simulink model "PHIL_testing"  (R2023b)
settings: Solver=ode4  StartTime=0.0  StopTime=inf  FixedStep=Ts  RelTol=1e-3
PostLoadFcn:
  | init;
InitFcn:
  | init;
values from neighbouring files (symbols this model uses):
  CURRENT_INPUT_OFFSET_PHA = 0    [init.m]
  CURRENT_INPUT_OFFSET_PHB = 0    [init.m]
  CURRENT_INPUT_OFFSET_PHC = 0    [init.m]
  CURRENT_INPUT_SCALE_PHA = 30    [init.m]
  CURRENT_INPUT_SCALE_PHB = 30    [init.m]
  CURRENT_INPUT_SCALE_PHC = 30    [init.m]
  ENABLE_PHA = 1    [init.m]
  ENABLE_PHB = 1    [init.m]
  ENABLE_PHC = 1    [init.m]
  FNOM = 60.0    (= 60)    [init.m]
  FREQUENCY = 60.0    (= 60)    [init.m]
  FREQUENCY_MAX_LIMIT = 66.0    (= 66)    [init.m]
  FREQUENCY_MIN_LIMIT = 56.0    (= 56)    [init.m]
  FRT_CONDITION = [1 1 1 0 ]    [init.m]
  FRT_END_TIMING = [0.2 0.3 0.4 0.5]    [init.m]
  FRT_START_TIMING = [0.1 0.2 0.3 0.4]    [init.m]
  FRT_VALUES = [59.0 56.0 55.0 33.0]    [init.m]
  MODE = 1    [init.m]
  PCRT_CONDITION = [ 0    1     0     2     0     3      0      4      0      4      0   ]    [init.m]
  PCRT_END_TIMING = [30.0 30.32 60.32 60.64 90.64 90.96 120.96 175.96 205.96 260.96 290.96]    [init.m]
  PCRT_START_TIMING = [ 0.0 30.0  30.32 60.32 60.64 90.64  90.96 120.96 175.96 205.96 260.96]    [init.m]
  PCRT_VALUES = [ 0.0 60.0   0.0  60.0   0.0  60.0    0.0   20.0    0.0  340.0    0.0 ]    [init.m]
  PHASE = [0.0 -120.0 120.0]    [init.m]
  PHNOM = [0 -120 120]    [init.m]
  Pnom = 5e3    (= 5000)    [init.m]
  RMS_ENABLE = 0    [init.m]
  ROCOF_ENABLE = 0    [init.m]
  ROCOF_INIT = 60    [init.m]
  ROCOF_VALUE = 3    [init.m]
  ROCOM_ENABLE = 1    [init.m]
  ROCOM_END_TIME = 100    [init.m]
  ROCOM_INIT = 1    [init.m]
  ROCOM_START_TIME = 0    [init.m]
  ROCOM_VALUE = 13.8    [init.m]
  Srated = 5e3    (= 5000)    [init.m]
  Ts = 40e-6    (= 4e-05)    [init.m]
  VNOM = 1.0    (= 1)    [init.m]
  VOLT_INPUT_OFFSET_PHA = 0    [init.m]
  VOLT_INPUT_OFFSET_PHB = 0    [init.m]
  VOLT_INPUT_OFFSET_PHC = 0    [init.m]
  VOLT_INPUT_SCALE_PHA = 100    [init.m]
  VOLT_INPUT_SCALE_PHB = 100    [init.m]
  VOLT_INPUT_SCALE_PHC = 100    [init.m]
  VOLT_OUTPUT_SCALE_PHA = 5.6    [init.m]
  VOLT_OUTPUT_SCALE_PHB = 5.6    [init.m]
  VOLT_OUTPUT_SCALE_PHC = 5.6    [init.m]
  VOLTAGE = [1.0 1.0 1.0]    [init.m]
  VOLTAGE_MAX_LIMIT = 1.1    [init.m]
  VOLTAGE_MIN_LIMIT = 0.0    (= 0)    [init.m]
  VRT_CONDITION = [0 1 0 1 0 1 0 1 -1 -1 -1 -1 -1 -1 -1 -1 -1 -1 -1 -1]+1    [init.m]
  VRT_END_TIMING = [0.2 0.3 0.4 0.5 0.6 0.7 0.8 0.9 1 1.1 1.2 1.3 1.4 1.5 1.6 1.7 1.8 1.9 2 2.1]    [init.m]
  VRT_PHA_ENABLE = 0    [init.m]
  VRT_PHB_ENABLE = 0    [init.m]
  VRT_PHC_ENABLE = 0    [init.m]
  VRT_START_TIMING = [0.1 0.2 0.3 0.4 0.5 0.6 0.7 0.8 0.9 1 0.1 0.2 0.3 0.4 0.5 0.6 0.7 0.8 0.9 1]    [init.m]
  VRT_VALUES = [1.2 0.94 0 0.5 0.7 0.88 0.94 0.88 0.94 1.1 1.2 0.94 0 0.5 0.7 0.88 0.94 0.88 0.94 1.1]    [init.m]
  WAV_ENABLE = 1    [init.m]
undefined symbols (not defined in the file or in its folder): another_event_name, DiscIntNeverNeededParam, EX, magnitude, my_event_name, TE0741_4, TwoSSS_AIO_CPWM
libraries: simulink x14, rtlab x6, simulink_extras x6, spsRMSLib x6, rtio_opalrt_common x4, eePowerMeasurement x3, rtio_opalrt_ml605ex1 x2, spsPLL3phLib x1, spspowerguiLib x1
(part 1 of 2)
settings Model: ARTEMISmethode_block_infos=$$__separator__$$  NumberOfSteps=10  Creator=DETLDAQ  LastModifiedBy=eudesjar
settings SolverCC: AlgebraicLoopSolver=TrustRegion
settings DataIOCC: LimitDataPoints=on  SaveFormat=Array  ReturnWorkspaceOutputs=off
settings OptimizationCC: BlockReduction=off  BooleanDataType=off  OptimizeBlockIOStorage=off  BufferReuse=off  GlobalBufferReuse=off  ExpressionFolding=off  LocalBlockOutputs=off  LifeSpan=inf  OptimizeDataStoreBuffers=off  BusAssignmentInplaceUpdate=off
settings DebuggingCC: SaveWithParameterizedLinksMsg=none  UnderspecifiedInitializationDetection=Classic  MergeDetectMultiDrivingBlocksExec=none  SignalResolutionControl=TryResolveAllWithWarning  MultiTaskDSMMsg=warning  MultiTaskCondExecSysMsg=none  UnconnectedInputMsg=warning  UnconnectedOutputMsg=warning  UnconnectedLineMsg=warning  StateNameClashWarn=warning  SFUnexpectedBacktrackingDiag=warning  SFNoUnconditionalDefaultTransitionDiag=warning  SFExecutionAtInitializationDiag=none  ArithmeticOperatorsInVariantConditions=warning
settings HardwareCC: ProdBitPerPointer=32  ProdBitPerSizeT=32  ProdBitPerPtrDiffT=32  ProdLargestAtomicFloat=None  ProdIntDivRoundTo=Undefined  ProdEndianess=Unspecified  ProdWordSize=32  ProdHWDeviceType=32-bit Generic  TargetBitPerPointer=64  TargetBitPerSizeT=64  TargetBitPerPtrDiffT=64  TargetLongLongMode=on  TargetIntDivRoundTo=Zero  TargetEndianess=LittleEndian  TargetWordSize=64  TargetHWDeviceType=MATLAB Host  ProdEqTarget=off
settings ModelReferenceCC: EnableRefExpFcnMdlSchedulingChecks=on  PropagateSignalLabelsOutOfModel=off
settings SFSimCC: SimUseLocalCustomCode=off  CustomCodeUndefinedFunction=UseInterfaceOnly
settings RTWCC: RTWUseLocalCustomCode=off  DLArmComputeVersion=19.05
settings CodeAppCC: StateflowObjectComments=on
settings GRTTargetCC: TargetLangStandard=C89/C90 (ANSI)
settings ConfigComp: CovMetricSettings=dw  CovSaveCumulativeToWorkspaceVar=on  CovSaveSingleToWorkspaceVar=on  CovExternalEMLEnable=off
settings SimscapeCC: SimscapeNormalizeSystem=off

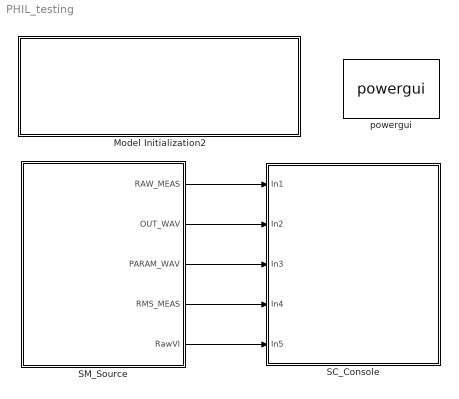
== system PHIL_testing ==
  Model Initialization2 : Subsystem  AncestorBlock=artemis/Tools /Misc/Model Initialization  mask(Model Functions){InitFcnX=init;, prel=off, posl=on, inif=on, strf=off}
      mask prompts: InitFcnX "Initialisation"; prel "Preload Function"; posl "PostLoad Function"; inif "InitFcn"; strf "StartFcn"
      mask init:
      | currentBlock = gcb;
      | root = bdroot(currentBlock);
      | 
      | if ~strcmp(get_param(root,'BlockDiagramType'),'library')
      |     if prel==1
      |         set_param(root, 'PreLoadFcn', InitFcnX);
      |     else
      |         set_param(root, 'PreLoadFcn', '');
      |     end
      |     if inif==1
      |         set_param(root, 'InitFcn', InitFcnX);
      |     else
      |         set_param(root, 'InitFcn', '');
      |     end
      |     if strf==1
      |         set_param(root, 'StartFcn', InitFcnX);
      |     else
      |         set_param(root, 'StartFcn', '');
      |     end
      |     if posl==1
      |         set_param(root, 'PostLoadFcn', InitFcnX);
      |     else
      |         set_param(root, 'PostLoadFcn', '');
      |     end
      | end
      | 
      | pos = get_param(currentBlock, 'Position');
      | width = pos(3) - pos(1); height = pos(4) - pos(2);
      | txt = [ upper(root) '\n' '- InitFcn. . . . . '  get_param(root, 'InitFcn') ];
      settings: CopyFcn=set_param(gcb,'LinkStatus','inactive')
      mask Display: text(5, height*0.5, txt, 'horizontalAlignment', 'left', 'verticalAlignment', 'middle') ;
  SC_Console : Subsystem
  SM_Source : Subsystem
  powergui : spspowerguiLib/powergui  Priority=1  SimulationMode=Discrete  SampleTime=Ts  frequency=60  Iterations=50  frequencyindice=0  Pbase=100e6  ErrMax=1e-4  UnitsV=kV  UnitsW=MW  buscounter=0  FunctionMessages=off  echomessages=off  EnableUseOfTLC=off  CurrentSourceSwitches=off  DisableSnubberDevices=off  DisableRonSwitches=off  DisableVfSwitches=off  DisplayEquations=off  AutomaticDiscreteSolvers=off  SolverType=Backward Euler  Interpol=off  ExternalGateDelay=off  methode=off  Ts=100  x0status=blocks  SPID=off  SwTol=0  HookPort=off  NonlinearTolerance=1e-4  nMaxIteration=100  ContinueOnMaxIteration=off  RestoreLinks=warning  ResistiveCurrentMeasurement=off  Frange=[0:2:500]  Ylog=off  Xlog=on  ShowGrid=off  save=off  variable=ZData  structure=0  ZoomFFT=off  StartTime=0.0  cycles=1  DisplayStyle=1  fundamental=60  FreqAxis=off  MaxFrequency=1000  frequencyindicesteady=1  RmsSteady=1  display=off
  wires:
  SM_Source/1(RAW_MEAS) -> SC_Console/1(In1)
  SM_Source/2(OUT_WAV) -> SC_Console/2(In2)
  SM_Source/3(PARAM_WAV) -> SC_Console/3(In3)
  SM_Source/4(RMS_MEAS) -> SC_Console/4(In4)
  SM_Source/5(RawVI) -> SC_Console/5(In5)

== system PHIL_testing/Model Initialization2 ==

== system PHIL_testing/SC_Console ==
  note: measurement after signal conditionning
  note: Input voltage and current after scaling and filtering
  note: Input voltage and current before scaling and filtering
  In1 : Inport
  In2 : Inport  Port=2
  In3 : Inport  Port=3
  In4 : Inport  Port=4
  In5 : Inport  Port=5
  Bus Selector : BusSelector  OutputSignals=voltage_pha,voltage_phb,voltage_phc,current_pha,current_phb,current_phc
  Bus Selector1 : BusSelector  OutputSignals=voltage_RMS,current_RMS,frequency,active_power,reactive_power,power_factor
  Bus Selector2 : BusSelector  OutputSignals=Raw Ia,Raw Ib,Raw Ic,Raw Va,Raw Vb,Raw Vc
  Display : Display
  Display1 : Display
  Display2 : Display
  Mux : Mux  Inputs=3
  Mux1 : Mux  Inputs=3
  OpComm : rtlab/OpComm  nbport=5  groupe_acq=1  subsys_rate=0  st=0  Synchronization=on  Interpolation=on  Threshold=1.0  Missed_Data=off  Sim_Time=off  Samples=off  dynSigOut=off  from_console=0  warning_done=off  writeOpCommFile=off  Offset=off
      settings: SourceProductName=RT-LAB
  Scope1 : Scope  NumInputPorts=6
  Scope2 : Scope  NumInputPorts=6
  Scope3 : Scope  NumInputPorts=3
  wires:
  In1/1 -> OpComm/1
  In2/1 -> OpComm/2
  In3/1 -> OpComm/3
  In4/1 -> OpComm/4
  OpComm/1 -> Bus Selector/1
  Bus Selector/1 -> Mux/1  "<voltage_pha>"
  Bus Selector/3 -> Mux/3  "<voltage_phc>"
  Mux/1 -> Scope3/1
  Mux1/1 -> Scope3/2
  Bus Selector/5 -> Mux1/2  "<current_phb>"
  Bus Selector/6 -> Mux1/3  "<current_phc>"
  Bus Selector/4 -> Mux1/1  "<current_pha>"
  OpComm/2 -> Scope3/3  "Output waveform"
  OpComm/3 -> Display/1  "waveform parameters"
  OpComm/4 -> Bus Selector1/1
  Bus Selector1/1 -> Display1/1, Scope1/1  "<voltage_RMS>"
  Bus Selector1/2 -> Display2/1, Scope1/2  "<current_RMS>"
  Bus Selector1/3 -> Scope1/3  "<frequency>"
  Bus Selector1/4 -> Scope1/4  "<active_power>"
  Bus Selector1/5 -> Scope1/5  "<reactive_power>"
  Bus Selector1/6 -> Scope1/6  "<power_factor>"
  In5/1 -> OpComm/5
  OpComm/5 -> Bus Selector2/1
  Bus Selector2/1 -> Scope2/1  "<Raw Ia>"
  Bus Selector2/2 -> Scope2/2  "<Raw Ib>"
  Bus Selector2/4 -> Scope2/4  "<Raw Va>"
  Bus Selector2/5 -> Scope2/5  "<Raw Vb>"
  Bus Selector2/6 -> Scope2/6  "<Raw Vc>"
  Bus Selector2/3 -> Scope2/3  "<Raw Ic>"
  Bus Selector/2 -> Mux/2  "<voltage_phb>"

== system PHIL_testing/SM_Source ==
  note: Phase, magnitude and frequency parameters of the waveform generator
  note: Voltage waveform sent as analog output
  note: RMS measurement after signal conditionning
  note: This subsytem includes a data acquistion system, a waveform generator and their control schemes
  note: This block is used to monitor the model's overruns with SVP
  note: Raw measurement before scaling and filtering
  note: Input connection with specific testbench Input blocks (needs to be redefined for new setup)
  note: Raw measurement after scaling and filtering
  note: output connection with specific testbench output blocks (needs to be redefined for new setup)
  Control : Subsystem
  InputConnections : Subsystem
  OpMonitor : rtlab/Monitoring/OpMonitor  compute_time=on  real_step=on  idle_time=on  nb_overruns=on  user_time=off  user_name=my_event_name,another_event_name
      settings: SourceProductName=RT-LAB
  OutputConnections : Subsystem
  Terminator : Terminator
  overruns : Gain
  RAW_MEAS : Outport  VectorParamsAs1DForOutWhenUnconnected=off
  OUT_WAV : Outport  Port=2  VectorParamsAs1DForOutWhenUnconnected=off
  PARAM_WAV : Outport  Port=3  VectorParamsAs1DForOutWhenUnconnected=off
  RMS_MEAS : Outport  Port=4  VectorParamsAs1DForOutWhenUnconnected=off
  RawVI : Outport  Port=5  VectorParamsAs1DForOutWhenUnconnected=off
  wires:
  InputConnections/1(RAW_MEAS (Nominal)) -> Control/1(RAW_MEAS (Nominal)), [RAW_MEAS]
  OpMonitor/4 -> overruns/1
  Control/1(OUT_WAV (PU)) -> [OUT_WAV], OutputConnections/1(OUT_WAV (PU))  "Output waveform"
  Control/2(PARAM_WAV (PU)) -> [PARAM_WAV]
  [PARAM_WAV] -> PARAM_WAV/1
  [RAW_MEAS] -> RAW_MEAS/1
  [OUT_WAV] -> OUT_WAV/1
  Control/3(RMS_MEAS) -> RMS_MEAS/1
  InputConnections/2(Out1) -> RawVI/1  "Raw measurements"
  overruns/1 -> Terminator/1

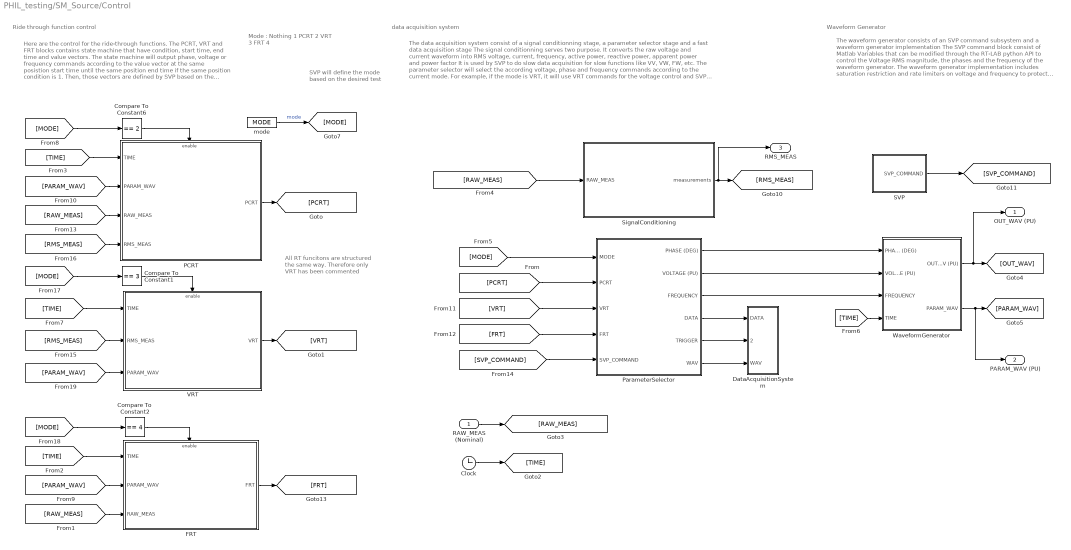
== system PHIL_testing/SM_Source/Control ==
  note: The waveform generator consists of an SVP command subsystem and a waveform generator implementation
      |
      | The SVP command block consist of Matlab Variables that can be modified through the RT-LAB python API to control the Voltage RMS magnitude, the phases and the frequency of the waveform generator.
      |
      | The waveform generator implementation includes saturation restriction and rate limiters on voltage and frequency to protect testbenches equipements. Those limits needs to be be setup properly in init.m. Then, after applying the different limitation, the voltage magnitude, phase and frequency is converted into a voltage waveform signal.
  note: The data acquisition system consist of a signal conditionning stage, a parameter selector stage and a fast data acquisition stage
      |
      | The signal conditionning serves two purpose.
      | It converts the raw voltage and current waveform into RMS voltage, current, frequency, active power, reactive power, apparent power and power factor
      | It is used by SVP to do slow data acquisition for slow functions like VV, VW, FW, etc.
      |
      | The parameter selector will select the according voltage, phase and frequency commands according to the current mode. For example, if the mode is VRT, it will use VRT commands for the voltage control and SVP commands for frequency and phase.
      |
      | The fast Data Acquisition System is used for fast recording since SVP is not fast enough to record transient behavior which is required for RT tests.
  note: All RT funcitons are structured the same way. Therefore only VRT has been commented
  note: SVP will define the mode based on the desired test
  note: Here are the control for the ride-through functions. The PCRT, VRT and FRT blocks contains state machine that have condition, start time, end time and value vectors. The state machine will output phase, voltage or frequency commands according to the value vector at the same posistion start time until the same position end time if the same position condition is 1.
      |
      | Then, those vectors are defined by SVP based on the script configuration.
  note: data acquisition system
  note: Waveform Generator
  note: Ride through function control
  note: Mode :
      |
      | Nothing
      | 1
      |
      | PCRT
      | 2
      |
      | VRT
      | 3
      |
      | FRT
      | 4
  RAW_MEAS (Nominal) : Inport
  Clock : Clock
  Compare To Constant1 : simulink/Logic and Bit Operations/Compare To Constant  relop===  const=3  OutDataTypeStr=boolean
  Compare To Constant2 : simulink/Logic and Bit Operations/Compare To Constant  relop===  const=4  OutDataTypeStr=boolean
  Compare To Constant6 : simulink/Logic and Bit Operations/Compare To Constant  relop===  const=2  OutDataTypeStr=boolean
  DataAcquisitionSystem : Subsystem
  FRT : Subsystem
  PCRT : Subsystem
  ParameterSelector : Subsystem
  SVP : Subsystem
  SignalConditioning : Subsystem
  VRT : Subsystem
  WaveformGenerator : Subsystem
  mode : Constant  Value=MODE
  OUT_WAV (PU) : Outport  VectorParamsAs1DForOutWhenUnconnected=off
  PARAM_WAV (PU) : Outport  Port=2  VectorParamsAs1DForOutWhenUnconnected=off
  RMS_MEAS : Outport  Port=3  VectorParamsAs1DForOutWhenUnconnected=off
  wires:
  mode/1 -> [MODE]  "mode"
  [RAW_MEAS] -> SignalConditioning/1(RAW_MEAS)
  [TIME] -> WaveformGenerator/4(TIME)
  ParameterSelector/5(TRIGGER) -> DataAcquisitionSystem/2(TRIGGER)
  ParameterSelector/1(PHASE (DEG)) -> WaveformGenerator/1(PHASE (DEG))
  [SVP_COMMAND] -> ParameterSelector/5(SVP_COMMAND)
  [MODE] -> ParameterSelector/1(MODE)
  Clock/1 -> [TIME]
  [MODE] -> Compare To Constant6/1
  [FRT] -> ParameterSelector/4(FRT)
  ParameterSelector/4(DATA) -> DataAcquisitionSystem/1(DATA)
  ParameterSelector/2(VOLTAGE (PU)) -> WaveformGenerator/2(VOLTAGE (PU))
  [VRT] -> ParameterSelector/3(VRT)
  WaveformGenerator/1(OUT_WAV (PU)) -> OUT_WAV (PU)/1, [OUT_WAV]
  [PCRT] -> ParameterSelector/2(PCRT)
  [RMS_MEAS] -> VRT/2(RMS_MEAS)
  ParameterSelector/3(FREQUENCY) -> WaveformGenerator/3(FREQUENCY)
  PCRT/1(PCRT) -> [PCRT]
  Compare To Constant6/1 -> PCRT/Enable
  [MODE] -> Compare To Constant1/1
  VRT/1(VRT) -> [VRT]
  [MODE] -> Compare To Constant2/1
  WaveformGenerator/2(PARAM_WAV) -> PARAM_WAV (PU)/1, [PARAM_WAV]
  Compare To Constant1/1 -> VRT/Enable
  [PARAM_WAV] -> VRT/3(PARAM_WAV)
  RAW_MEAS (Nominal)/1 -> [RAW_MEAS]
  [TIME] -> VRT/1(TIME)
  [TIME] -> FRT/1(TIME)
  Compare To Constant2/1 -> FRT/Enable
  FRT/1(FRT) -> [FRT]
  [PARAM_WAV] -> FRT/2(PARAM_WAV)
  [RAW_MEAS] -> FRT/3(RAW_MEAS)
  ParameterSelector/6(WAV) -> DataAcquisitionSystem/3(WAV)
  SignalConditioning/1(measurements) -> RMS_MEAS/1, [RMS_MEAS]
  SVP/1(SVP_COMMAND) -> [SVP_COMMAND]
  [RMS_MEAS] -> PCRT/4(RMS_MEAS)
  [PARAM_WAV] -> PCRT/2(PARAM_WAV)
  [RAW_MEAS] -> PCRT/3(RAW_MEAS)
  [TIME] -> PCRT/1(TIME)

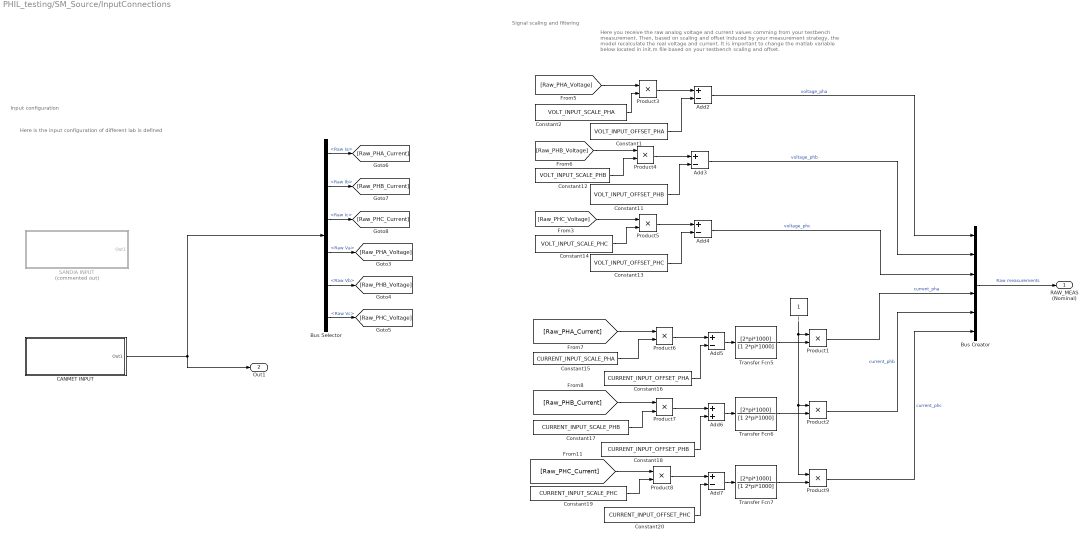
== system PHIL_testing/SM_Source/InputConnections ==
  note: Here is the input configuration of different lab is defined
  note: Input configuration
  note: Here you receive the raw analog voltage and current values comming from your testbench measurement. Then, based on scaling and offset induced by your measurement strategy, the model recalculate the real voltage and current.
      |
      | It is important to change the matlab variable below located in init.m file based on your testbench scaling and offset.
  note: Signal scaling and filtering
  Add{2..5,7} (5 alike) : Sum  Inputs=+-
  Add6 : Sum
  Bus Creator : BusCreator  Inputs=6
  Bus Selector : BusSelector  OutputSignals=Raw Ia,Raw Ib,Raw Ic,Raw Va,Raw Vb,Raw Vc
  CANMET INPUT : Subsystem
  Constant1 : Constant  Value=VOLT_INPUT_OFFSET_PHA
  Constant11 : Constant  Value=VOLT_INPUT_OFFSET_PHB
  Constant12 : Constant  Value=VOLT_INPUT_SCALE_PHB
  Constant13 : Constant  Value=VOLT_INPUT_OFFSET_PHC
  Constant14 : Constant  Value=VOLT_INPUT_SCALE_PHC
  Constant15 : Constant  Value=CURRENT_INPUT_SCALE_PHA
  Constant16 : Constant  Value=CURRENT_INPUT_OFFSET_PHA
  Constant17 : Constant  Value=CURRENT_INPUT_SCALE_PHB
  Constant18 : Constant  Value=CURRENT_INPUT_OFFSET_PHB
  Constant19 : Constant  Value=CURRENT_INPUT_SCALE_PHC
  Constant2 : Constant  Value=VOLT_INPUT_SCALE_PHA
  Constant20 : Constant  Value=CURRENT_INPUT_OFFSET_PHC
  I : Constant
  Product{1..9} (9 alike) : Product
  SANDIA INPUT : Subsystem  Commented=on
  Transfer Fcn5 : TransferFcn  Numerator=[2*pi*1000]  Denominator=[1 2*pi*1000]
  Transfer Fcn6 : TransferFcn  Numerator=[2*pi*1000]  Denominator=[1 2*pi*1000]
  Transfer Fcn7 : TransferFcn  Numerator=[2*pi*1000]  Denominator=[1 2*pi*1000]
  RAW_MEAS (Nominal) : Outport  VectorParamsAs1DForOutWhenUnconnected=off
  Out1 : Outport  Port=2  VectorParamsAs1DForOutWhenUnconnected=off
  wires:
  [Raw_PHB_Current] -> Product7/1
  Product6/1 -> Add5/1
  Constant17/1 -> Product7/2
  I/1 -> Product2/1, Product9/1, Product1/1
  Transfer Fcn6/1 -> Product2/2
  Constant14/1 -> Product5/2
  Constant13/1 -> Add4/2
  [Raw_PHB_Voltage] -> Product4/1
  Product8/1 -> Add7/1
  Product5/1 -> Add4/1
  Constant15/1 -> Product6/2
  [Raw_PHC_Voltage] -> Product5/1
  Constant20/1 -> Add7/2
  Add6/1 -> Transfer Fcn6/1
  Add5/1 -> Transfer Fcn5/1
  Product7/1 -> Add6/1
  [Raw_PHA_Voltage] -> Product3/1
  Constant18/1 -> Add6/2
  [Raw_PHA_Current] -> Product6/1
  Transfer Fcn7/1 -> Product9/2
  [Raw_PHC_Current] -> Product8/1
  Add7/1 -> Transfer Fcn7/1
  Constant16/1 -> Add5/2
  Transfer Fcn5/1 -> Product1/2
  Product4/1 -> Add3/1
  Product3/1 -> Add2/1
  Constant19/1 -> Product8/2
  Add2/1 -> Bus Creator/1  "voltage_pha"
  Add3/1 -> Bus Creator/2  "voltage_phb"
  Add4/1 -> Bus Creator/3  "voltage_phc"
  Product1/1 -> Bus Creator/4  "current_pha"
  Product2/1 -> Bus Creator/5  "current_phb"
  Product9/1 -> Bus Creator/6  "current_phc"
  Bus Creator/1 -> RAW_MEAS (Nominal)/1  "Raw measurements"
  Constant2/1 -> Product3/2
  Constant11/1 -> Add3/2
  Constant12/1 -> Product4/2
  Constant1/1 -> Add2/2
  Bus Selector/1 -> [Raw_PHA_Current]  "<Raw Ia>"
  Bus Selector/2 -> [Raw_PHB_Current]  "<Raw Ib>"
  Bus Selector/3 -> [Raw_PHC_Current]  "<Raw Ic>"
  Bus Selector/4 -> [Raw_PHA_Voltage]  "<Raw Va>"
  Bus Selector/5 -> [Raw_PHB_Voltage]  "<Raw Vb>"
  Bus Selector/6 -> [Raw_PHC_Voltage]  "<Raw Vc>"
  CANMET INPUT/1(Out1) -> Out1/1, Bus Selector/1

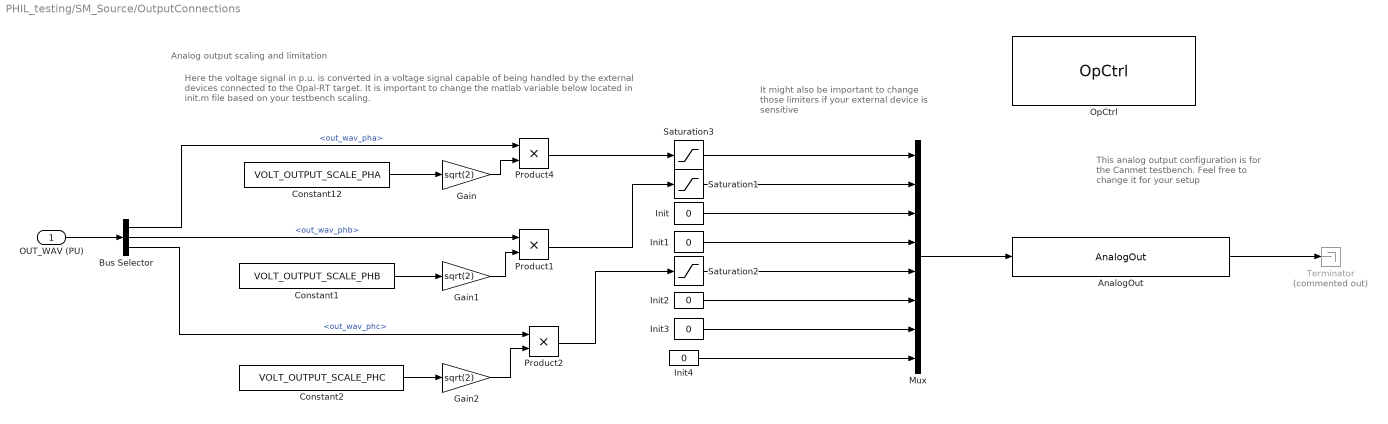
== system PHIL_testing/SM_Source/OutputConnections ==
  note: This analog output configuration is for the Canmet testbench. Feel free to change it for your setup
  note: It might also be important to change those limiters if your external device is sensitive
  note: Here the voltage signal in p.u. is converted in a voltage signal capable of being handled by the external devices connected to the Opal-RT target.
      |
      | It is important to change the matlab variable below located in init.m file based on your testbench scaling.
  note: Analog output scaling and limitation
  OUT_WAV (PU) : Inport
  AnalogOut : rtio_opalrt_common/AnalogOut  CtrlName='OpCtrl'  portNb=7  FcnNos=Slot 2 Module B Subsection 1  size=16  maxcount=8  count=8  numchan=8  israngeinput=off  voltagerange=[-16 ... 16]  slot=1  side=1  mismatch=0  slotside=Slot_2_Module_B
      settings: AttributesFormatString=%<CtrlName>  SourceProductName=RT-LAB I/O
  Bus Selector : BusSelector  OutputSignals=out_wav_pha,out_wav_phb,out_wav_phc
  Constant1 : Constant  Value=VOLT_OUTPUT_SCALE_PHB
  Constant12 : Constant  Value=VOLT_OUTPUT_SCALE_PHA
  Constant2 : Constant  Value=VOLT_OUTPUT_SCALE_PHC
  Gain : Gain  Gain=sqrt(2)
  Gain1 : Gain  Gain=sqrt(2)
  Gain2 : Gain  Gain=sqrt(2)
  Init{,1..4} (5 alike) : Constant  Value=0
  Mux : Mux  Inputs=8
  OpCtrl : rtio_opalrt_common/OpCtrl  CtrlName='OpCtrl'  boardid=0  BitstreamFilename=TE0741_4-EX-0001-3_5_0_817-TwoSSS_AIO_CPWM-04-01.bin  numconfig=-1  mode=Master  externalClock=off  decimRtsi=0  calibIO=off  SampleTime=0  loadinport=-1  BoardType=TE0741  SecondaryPresent=off  sync_type=Optical fiber  scope_enable=off  fsdFileName=TE0741_4-EX-0001-3_5_0_817-TwoSSS_AIO_CPWM-04-01.fsd  mismatch_disable=on
      settings: SourceProductName=RT-LAB I/O
  Product1 : Product
  Product2 : Product
  Product4 : Product
  Saturation1 : Saturate  UpperLimit=15  LowerLimit=-15
  Saturation2 : Saturate  UpperLimit=15  LowerLimit=-15
  Saturation3 : Saturate  UpperLimit=15  LowerLimit=-15
  Terminator : Terminator  Commented=on
  wires:
  OUT_WAV (PU)/1 -> Bus Selector/1
  Product1/1 -> Saturation1/1
  Product2/1 -> Saturation2/1
  Product4/1 -> Saturation3/1
  Constant12/1 -> Gain/1
  Bus Selector/1 -> Product4/1  "<out_wav_pha>"
  Constant1/1 -> Gain1/1
  Bus Selector/2 -> Product1/1  "<out_wav_phb>"
  Constant2/1 -> Gain2/1
  Bus Selector/3 -> Product2/1  "<out_wav_phc>"
  Saturation2/1 -> Mux/5
  Saturation3/1 -> Mux/1
  Saturation1/1 -> Mux/2
  Mux/1 -> AnalogOut/1
  Init/1 -> Mux/3
  Init1/1 -> Mux/4
  Init2/1 -> Mux/6
  Init3/1 -> Mux/7
  Init4/1 -> Mux/8
  AnalogOut/1 -> Terminator/1
  Gain/1 -> Product4/2
  Gain1/1 -> Product1/2
  Gain2/1 -> Product2/2

== system PHIL_testing/SM_Source/Control/DataAcquisitionSystem ==
  note: There is two types of recording depending on the RT function requirements either RMS or waveform data acquisition
  note: Here the RT state machine will send a trigger signal to start the recording
  DATA : Inport
  TRIGGER : Inport  Port=2
  WAV : Inport  Port=3
  Compare To Constant1 : simulink/Logic and Bit Operations/Compare To Constant  relop===  const=1  OutDataTypeStr=boolean
  Compare To Constant2 : simulink/Logic and Bit Operations/Compare To Constant  relop===  const=1  OutDataTypeStr=boolean
  Constant : Constant  Value=RMS_ENABLE
  Constant1 : Constant  Value=WAV_ENABLE
  OpTrigger : rtlab/DataLogging/OpTrigger  Trig_Type=TRIGGER SIGNAL >= TRIGGER LEVEL  Trig_Offset=-(1/Ts)  Acq_Group=28
      settings: SourceProductName=RT-LAB
  OpTrigger1 : rtlab/DataLogging/OpTrigger  Trig_Type=TRIGGER SIGNAL >= TRIGGER LEVEL  Trig_Offset=0  Acq_Group=27
      settings: SourceProductName=RT-LAB
  Subsystem : Subsystem
  Subsystem1 : Subsystem
  TRIGGER_STATUS : Gain
  TRIGGER_STATUS1 : Gain
  Terminator2 : Terminator
  Terminator3 : Terminator
  Trigger_level : Constant
  wires:
  OpTrigger/1 -> TRIGGER_STATUS/1
  Trigger_level/1 -> OpTrigger/2, OpTrigger1/2
  TRIGGER_STATUS/1 -> Terminator2/1
  TRIGGER_STATUS1/1 -> Terminator3/1
  OpTrigger1/1 -> TRIGGER_STATUS1/1
  TRIGGER/1 -> OpTrigger1/1, OpTrigger/1
  DATA/1 -> Subsystem/1(In1)
  Constant/1 -> Compare To Constant1/1
  Compare To Constant1/1 -> Subsystem/Enable
  Constant1/1 -> Compare To Constant2/1
  Compare To Constant2/1 -> Subsystem1/Enable
  WAV/1 -> Subsystem1/1(In1)

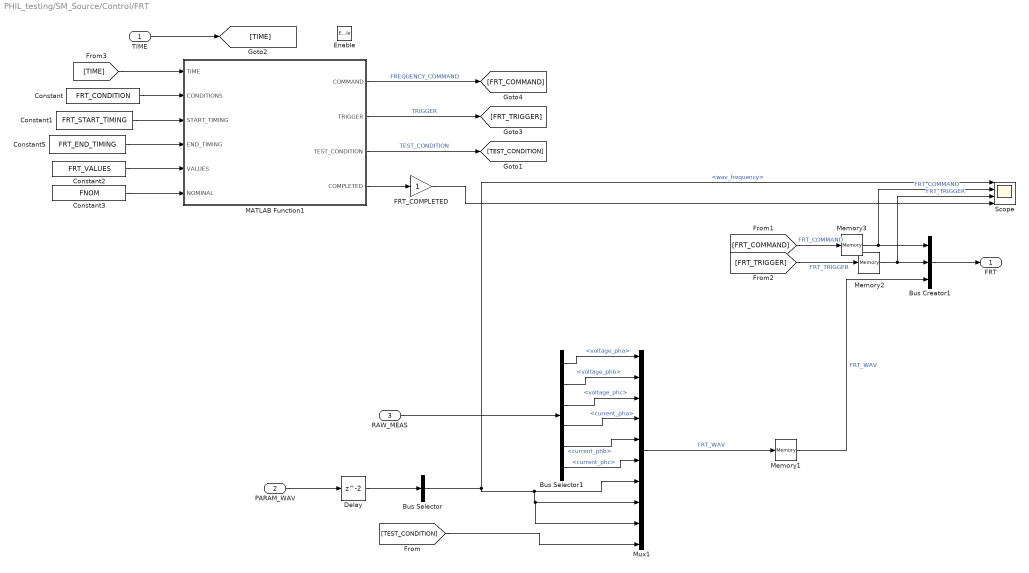
== system PHIL_testing/SM_Source/Control/FRT ==
  TIME : Inport
  PARAM_WAV : Inport  Port=2
  RAW_MEAS : Inport  Port=3
  Enable : EnablePort
  Bus Creator1 : BusCreator  Inputs=3
  Bus Selector : BusSelector  OutputSignals=wav_frequency
  Bus Selector1 : BusSelector  OutputSignals=voltage_pha,voltage_phb,voltage_phc,current_pha,current_phb,current_phc
  Constant : Constant  Value=FRT_CONDITION
  Constant1 : Constant  Value=FRT_START_TIMING
  Constant2 : Constant  Value=FRT_VALUES
  Constant3 : Constant  Value=FNOM
  Constant5 : Constant  Value=FRT_END_TIMING
  Delay : Delay
  FRT_COMPLETED : Gain
  MATLAB Function1 : MATLAB Function  TreatAsAtomicUnit=on
  Memory1 : Memory  InheritSampleTime=on  LinearizeMemory=on
  Memory2 : Memory  InheritSampleTime=on  LinearizeMemory=on
  Memory3 : Memory  InitialCondition=FNOM  InheritSampleTime=on  LinearizeMemory=on
  Mux1 : Mux  Inputs=10
  Scope : Scope  NumInputPorts=4
  FRT : Outport
  wires:
  Mux1/1 -> Memory1/1  "FRT_WAV"
  MATLAB Function1/1(COMMAND) -> [FRT_COMMAND]  "FREQUENCY_COMMAND"
  MATLAB Function1/3(TEST_CONDITION) -> [TEST_CONDITION]  "TEST_CONDITION"
  [TIME] -> MATLAB Function1/1(TIME)
  [FRT_TRIGGER] -> Memory2/1  "FRT_TRIGGER"
  Constant/1 -> MATLAB Function1/2(CONDITIONS)
  TIME/1 -> [TIME]
  Constant2/1 -> MATLAB Function1/5(VALUES)
  Constant5/1 -> MATLAB Function1/4(END_TIMING)
  MATLAB Function1/2(TRIGGER) -> [FRT_TRIGGER]  "TRIGGER"
  PARAM_WAV/1 -> Delay/1
  Bus Creator1/1 -> FRT/1
  MATLAB Function1/4(COMPLETED) -> FRT_COMPLETED/1
  Constant1/1 -> MATLAB Function1/3(START_TIMING)
  [FRT_COMMAND] -> Memory3/1  "FRT_COMMAND"
  [TEST_CONDITION] -> Mux1/10
  Delay/1 -> Bus Selector/1
  Bus Selector/1 -> Scope/1, Mux1/9, Mux1/8, Mux1/7  "<wav_frequency>"
  RAW_MEAS/1 -> Bus Selector1/1
  Bus Selector1/1 -> Mux1/1  "<voltage_pha>"
  Bus Selector1/2 -> Mux1/2  "<voltage_phb>"
  Bus Selector1/3 -> Mux1/3  "<voltage_phc>"
  Constant3/1 -> MATLAB Function1/6(NOMINAL)
  FRT_COMPLETED/1 -> Scope/4
  Bus Selector1/4 -> Mux1/4  "<current_pha>"
  Bus Selector1/5 -> Mux1/5  "<current_phb>"
  Bus Selector1/6 -> Mux1/6  "<current_phc>"
  Memory1/1 -> Bus Creator1/3  "FRT_WAV"
  Memory2/1 -> Scope/3, Bus Creator1/2  "FRT_TRIGGER"
  Memory3/1 -> Scope/2, Bus Creator1/1  "FRT_COMMAND"

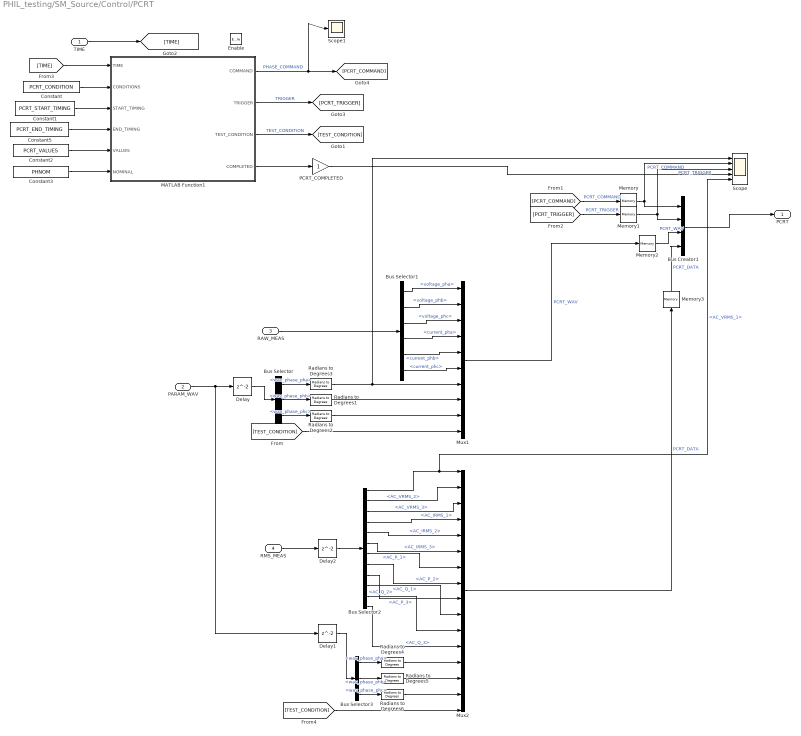
== system PHIL_testing/SM_Source/Control/PCRT ==
  TIME : Inport
  PARAM_WAV : Inport  Port=2
  RAW_MEAS : Inport  Port=3
  RMS_MEAS : Inport  Port=4
  Enable : EnablePort
  Bus Creator1 : BusCreator  Inputs=4
  Bus Selector : BusSelector  OutputSignals=wav_phase_pha,wav_phase_phb,wav_phase_phc
  Bus Selector1 : BusSelector  OutputSignals=voltage_pha,voltage_phb,voltage_phc,current_pha,current_phb,current_phc
  Bus Selector2 : BusSelector  OutputSignals=voltage_RMS.AC_VRMS_1,voltage_RMS.AC_VRMS_2,voltage_RMS.AC_VRMS_3,current_RMS.AC_IRMS_1,current_RMS.AC_IRMS_2,current_RMS.AC_IRMS_3,active_power.AC_P_1,active_power.AC_P_2,active_power.AC_P_3,reactive_power.AC_Q_1,reactive_power.AC_Q_2,reactive_power.AC_Q_3
  Bus Selector3 : BusSelector  OutputSignals=wav_phase_pha,wav_phase_phb,wav_phase_phc
  Constant : Constant  Value=PCRT_CONDITION
  Constant1 : Constant  Value=PCRT_START_TIMING
  Constant2 : Constant  Value=PCRT_VALUES
  Constant3 : Constant  Value=PHNOM
  Constant5 : Constant  Value=PCRT_END_TIMING
  Delay : Delay
  Delay1 : Delay
  Delay2 : Delay
  MATLAB Function1 : MATLAB Function  TreatAsAtomicUnit=on
  Memory : Memory  InitialCondition=PHNOM  InheritSampleTime=on  LinearizeMemory=on
  Memory1 : Memory  InheritSampleTime=on  LinearizeMemory=on
  Memory2 : Memory  InheritSampleTime=on  LinearizeMemory=on
  Memory3 : Memory  InheritSampleTime=on  LinearizeMemory=on
  Mux1 : Mux  Inputs=10
  Mux2 : Mux  Inputs=16
  PCRT_COMPLETED : Gain
  Radians to Degrees{1..6} (6 alike) : simulink_extras/Transformations/Radians to Degrees
  Scope : Scope  NumInputPorts=5
  Scope1 : Scope
  PCRT : Outport
  wires:
  Mux1/1 -> Memory2/1  "PCRT_WAV"
  MATLAB Function1/1(COMMAND) -> Scope1/1, [PCRT_COMMAND]  "PHASE_COMMAND"
  MATLAB Function1/3(TEST_CONDITION) -> [TEST_CONDITION]  "TEST_CONDITION"
  [TIME] -> MATLAB Function1/1(TIME)
  [PCRT_TRIGGER] -> Memory1/1  "PCRT_TRIGGER"
  Constant/1 -> MATLAB Function1/2(CONDITIONS)
  TIME/1 -> [TIME]
  Constant2/1 -> MATLAB Function1/5(VALUES)
  Constant5/1 -> MATLAB Function1/4(END_TIMING)
  MATLAB Function1/2(TRIGGER) -> [PCRT_TRIGGER]  "TRIGGER"
  MATLAB Function1/4(COMPLETED) -> PCRT_COMPLETED/1
  Constant1/1 -> MATLAB Function1/3(START_TIMING)
  [PCRT_COMMAND] -> Memory/1  "PCRT_COMMAND"
  [TEST_CONDITION] -> Mux1/10
  Delay/1 -> Bus Selector/1
  Bus Selector/1 -> Radians to Degrees3/1  "<wav_phase_pha>"
  RAW_MEAS/1 -> Bus Selector1/1
  Bus Selector1/1 -> Mux1/1  "<voltage_pha>"
  Bus Selector1/2 -> Mux1/2  "<voltage_phb>"
  Bus Selector1/3 -> Mux1/3  "<voltage_phc>"
  Constant3/1 -> MATLAB Function1/6(NOMINAL)
  PCRT_COMPLETED/1 -> Scope/4
  Bus Selector1/4 -> Mux1/4  "<current_pha>"
  Bus Selector1/5 -> Mux1/5  "<current_phb>"
  Bus Selector1/6 -> Mux1/6  "<current_phc>"
  Bus Creator1/1 -> PCRT/1
  Memory/1 -> Scope/2, Bus Creator1/1  "PCRT_COMMAND"
  Memory1/1 -> Scope/3, Bus Creator1/2  "PCRT_TRIGGER"
  Memory2/1 -> Bus Creator1/3  "PCRT_WAV"
  Bus Selector/2 -> Radians to Degrees1/1  "<wav_phase_phb>"
  Bus Selector/3 -> Radians to Degrees2/1  "<wav_phase_phc>"
  Radians to Degrees3/1 -> Scope/1, Mux1/7
  Radians to Degrees1/1 -> Mux1/8
  Radians to Degrees2/1 -> Mux1/9
  Bus Selector2/10 -> Mux2/10  "<AC_Q_1>"
  Bus Selector2/8 -> Mux2/8  "<AC_P_2>"
  Bus Selector2/11 -> Mux2/11  "<AC_Q_2>"
  Bus Selector2/12 -> Mux2/12  "<AC_Q_3>"
  Bus Selector3/2 -> Radians to Degrees5/1  "<wav_phase_phb>"
  Bus Selector2/9 -> Mux2/9  "<AC_P_3>"
  PARAM_WAV/1 -> Delay/1, Delay1/1
  Bus Selector3/3 -> Radians to Degrees6/1  "<wav_phase_phc>"
  Bus Selector3/1 -> Radians to Degrees4/1  "<wav_phase_pha>"
  Bus Selector2/7 -> Mux2/7  "<AC_P_1>"
  Bus Selector2/6 -> Mux2/6  "<AC_IRMS_3>"
  Bus Selector2/5 -> Mux2/5  "<AC_IRMS_2>"
  Bus Selector2/2 -> Mux2/2  "<AC_VRMS_2>"
  Delay2/1 -> Bus Selector2/1
  Mux2/1 -> Memory3/1  "PCRT_DATA"
  Bus Selector2/3 -> Mux2/3  "<AC_VRMS_3>"
  Bus Selector2/1 -> Scope/5, Mux2/1  "<AC_VRMS_1>"
  Bus Selector2/4 -> Mux2/4  "<AC_IRMS_1>"
  [TEST_CONDITION] -> Mux2/16
  Delay1/1 -> Bus Selector3/1
  RMS_MEAS/1 -> Delay2/1
  Radians to Degrees6/1 -> Mux2/15
  Radians to Degrees5/1 -> Mux2/14
  Radians to Degrees4/1 -> Mux2/13
  Memory3/1 -> Bus Creator1/4  "PCRT_DATA"

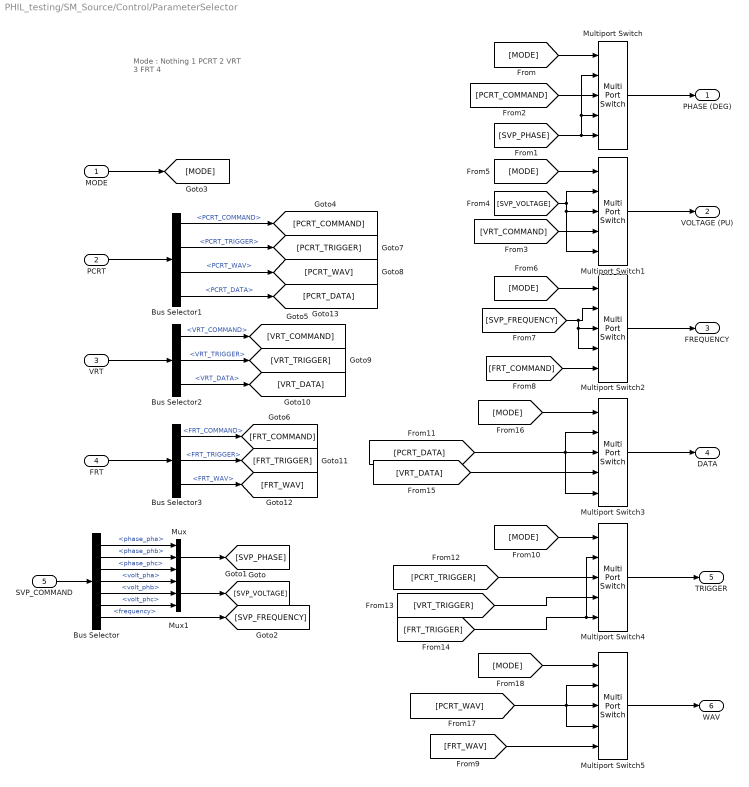
== system PHIL_testing/SM_Source/Control/ParameterSelector ==
  note: Mode :
      |
      | Nothing
      | 1
      |
      | PCRT
      | 2
      |
      | VRT
      | 3
      |
      | FRT
      | 4
  MODE : Inport
  PCRT : Inport  Port=2
  VRT : Inport  Port=3
  FRT : Inport  Port=4
  SVP_COMMAND : Inport  Port=5
  Bus Selector : BusSelector  OutputSignals=phase_pha,phase_phb,phase_phc,volt_pha,volt_phb,volt_phc,frequency
  Bus Selector1 : BusSelector  OutputSignals=PCRT_COMMAND,PCRT_TRIGGER,PCRT_WAV,PCRT_DATA
  Bus Selector2 : BusSelector  OutputSignals=VRT_COMMAND,VRT_TRIGGER,VRT_DATA
  Bus Selector3 : BusSelector  OutputSignals=FRT_COMMAND,FRT_TRIGGER,FRT_WAV
  Multiport Switch{,1..5} (6 alike) : MultiPortSwitch  Inputs=4  SaturateOnIntegerOverflow=off  InputSameDT=off
  Mux : Mux  Inputs=3
  Mux1 : Mux  Inputs=3
  PHASE (DEG) : Outport
  VOLTAGE (PU) : Outport  Port=2
  FREQUENCY : Outport  Port=3
  DATA : Outport  Port=4
  TRIGGER : Outport  Port=5
  WAV : Outport  Port=6
  wires:
  SVP_COMMAND/1 -> Bus Selector/1
  Bus Selector/2 -> Mux/2  "<phase_phb>"
  Bus Selector/1 -> Mux/1  "<phase_pha>"
  Bus Selector/3 -> Mux/3  "<phase_phc>"
  Bus Selector/4 -> Mux1/1  "<volt_pha>"
  Bus Selector/5 -> Mux1/2  "<volt_phb>"
  Bus Selector/6 -> Mux1/3  "<volt_phc>"
  Mux/1 -> [SVP_PHASE]
  Mux1/1 -> [SVP_VOLTAGE]
  Bus Selector/7 -> [SVP_FREQUENCY]  "<frequency>"
  MODE/1 -> [MODE]
  [MODE] -> Multiport Switch/1
  [PCRT_COMMAND] -> Multiport Switch/3
  [SVP_PHASE] -> Multiport Switch/2, Multiport Switch/4, Multiport Switch/5
  Multiport Switch/1 -> PHASE (DEG)/1
  Multiport Switch1/1 -> VOLTAGE (PU)/1
  Multiport Switch2/1 -> FREQUENCY/1
  [VRT_COMMAND] -> Multiport Switch1/4
  [SVP_VOLTAGE] -> Multiport Switch1/3, Multiport Switch1/5, Multiport Switch1/2
  [MODE] -> Multiport Switch1/1
  [MODE] -> Multiport Switch2/1
  [SVP_FREQUENCY] -> Multiport Switch2/3, Multiport Switch2/4, Multiport Switch2/2
  [FRT_COMMAND] -> Multiport Switch2/5
  PCRT/1 -> Bus Selector1/1
  Bus Selector1/1 -> [PCRT_COMMAND]  "<PCRT_COMMAND>"
  Bus Selector1/2 -> [PCRT_TRIGGER]  "<PCRT_TRIGGER>"
  Bus Selector1/3 -> [PCRT_WAV]  "<PCRT_WAV>"
  [VRT_DATA] -> Multiport Switch3/4
  Multiport Switch4/1 -> TRIGGER/1
  VRT/1 -> Bus Selector2/1
  Bus Selector2/1 -> [VRT_COMMAND]  "<VRT_COMMAND>"
  Bus Selector2/2 -> [VRT_TRIGGER]  "<VRT_TRIGGER>"
  Bus Selector2/3 -> [VRT_DATA]  "<VRT_DATA>"
  FRT/1 -> Bus Selector3/1
  Bus Selector3/1 -> [FRT_COMMAND]  "<FRT_COMMAND>"
  Bus Selector3/2 -> [FRT_TRIGGER]  "<FRT_TRIGGER>"
  Bus Selector3/3 -> [FRT_WAV]  "<FRT_WAV>"
  [MODE] -> Multiport Switch4/1
  [PCRT_TRIGGER] -> Multiport Switch4/3
  [PCRT_DATA] -> Multiport Switch3/2, Multiport Switch3/5, Multiport Switch3/3
  [VRT_TRIGGER] -> Multiport Switch4/4
  [FRT_TRIGGER] -> Multiport Switch4/2, Multiport Switch4/5
  [PCRT_WAV] -> Multiport Switch5/4, Multiport Switch5/2, Multiport Switch5/3
  Bus Selector1/4 -> [PCRT_DATA]  "<PCRT_DATA>"
  [FRT_WAV] -> Multiport Switch5/5
  Multiport Switch3/1 -> DATA/1
  [MODE] -> Multiport Switch3/1
  [MODE] -> Multiport Switch5/1
  Multiport Switch5/1 -> WAV/1

== system PHIL_testing/SM_Source/Control/SVP ==
  Bus Creator : BusCreator  Inputs=7
  Constant1 : Constant  Value=PHASE
  Constant2 : Constant  Value=VOLTAGE
  Constant3 : Constant  Value=FREQUENCY
  Demux : Demux  Outputs=3
  Demux1 : Demux  Outputs=3
  Gain{,1..3} (4 alike) : Gain
  SVP_COMMAND : Outport  VectorParamsAs1DForOutWhenUnconnected=off
  wires:
  Bus Creator/1 -> SVP_COMMAND/1
  Constant1/1 -> Demux/1
  Demux/1 -> Bus Creator/1  "phase_pha"
  Demux/2 -> Bus Creator/2  "phase_phb"
  Demux/3 -> Bus Creator/3  "phase_phc"
  Gain2/1 -> Bus Creator/6  "volt_phc"
  Gain1/1 -> Bus Creator/5  "volt_phb"
  Gain/1 -> Bus Creator/4  "volt_pha"
  Demux1/3 -> Gain2/1  "volt_phc"
  Demux1/2 -> Gain1/1  "volt_phb"
  Demux1/1 -> Gain/1  "volt_pha"
  Gain3/1 -> Bus Creator/7  "frequency"
  Constant2/1 -> Demux1/1
  Constant3/1 -> Gain3/1  "frequency"

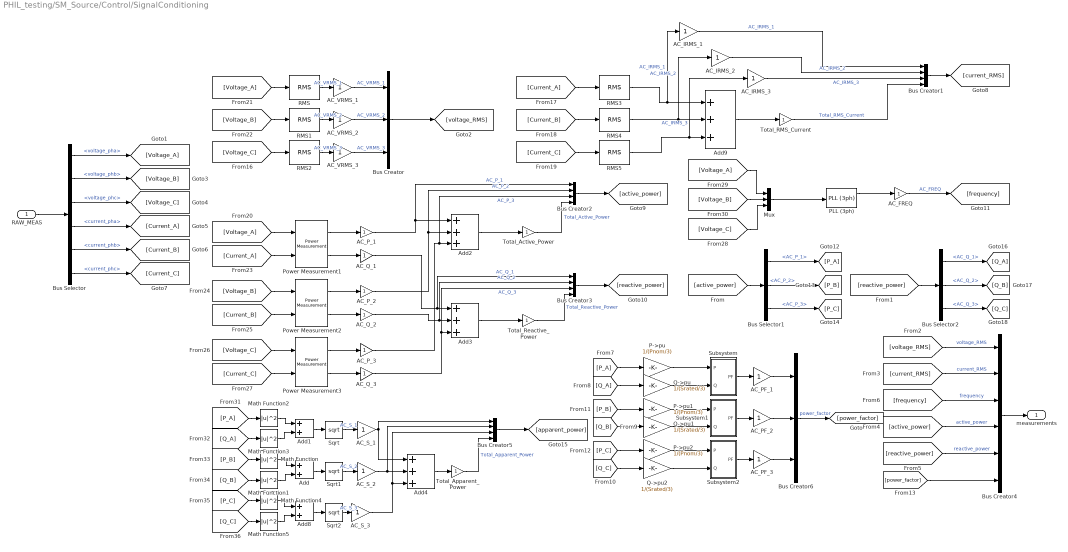
== system PHIL_testing/SM_Source/Control/SignalConditioning ==
  RAW_MEAS : Inport
  AC_FREQ : Gain
  AC_IRMS_1 : Gain
  AC_IRMS_2 : Gain
  AC_IRMS_3 : Gain
  AC_PF_1 : Gain
  AC_PF_2 : Gain
  AC_PF_3 : Gain
  AC_P_1 : Gain
  AC_P_2 : Gain
  AC_P_3 : Gain
  AC_Q_1 : Gain
  AC_Q_2 : Gain
  AC_Q_3 : Gain
  AC_S_1 : Gain
  AC_S_2 : Gain
  AC_S_3 : Gain
  AC_VRMS_1 : Gain
  AC_VRMS_2 : Gain
  AC_VRMS_3 : Gain
  Add : Sum
  Add1 : Sum
  Add{2..4,9} (4 alike) : Sum  Inputs=+++
  Add8 : Sum
  Bus Creator : BusCreator  Inputs=3
  Bus Creator{1..3,5} (4 alike) : BusCreator  Inputs=4
  Bus Creator4 : BusCreator  Inputs=6
  Bus Creator6 : BusCreator  Inputs=3
  Bus Selector : BusSelector  OutputSignals=voltage_pha,voltage_phb,voltage_phc,current_pha,current_phb,current_phc
  Bus Selector1 : BusSelector  OutputSignals=AC_P_1,AC_P_2,AC_P_3
  Bus Selector2 : BusSelector  OutputSignals=AC_Q_1,AC_Q_2,AC_Q_3
  Math Function{,1..5} (6 alike) : Math  Operator=magnitude^2  SignedPower=on
  Mux : Mux  Inputs=3
  P->pu : Gain  Gain=1/(Pnom/3)
  P->pu1 : Gain  Gain=1/(Pnom/3)
  P->pu2 : Gain  Gain=1/(Pnom/3)
  PLL (3ph) : spsPLL3phLib/PLL (3ph)  Fmin=50  Par_Init=[0, 60]  ParK=[180, 3200, 1]  TcD=Ts  MaxRateChangeFreq=5  FilterCutOffFreq=25  Ts=Ts  AGC=on
  Power Measurement1 : eePowerMeasurement/Power Measurement  LabelModeActiveChoice=Discrete  F=60  K=[1]  Ts=Ts
  Power Measurement2 : eePowerMeasurement/Power Measurement  LabelModeActiveChoice=Discrete  F=60  K=[1]  Ts=Ts
  Power Measurement3 : eePowerMeasurement/Power Measurement  LabelModeActiveChoice=Discrete  F=60  K=[1]  Ts=Ts
  Q->pu : Gain  Gain=1/(Srated/3)
  Q->pu1 : Gain  Gain=1/(Srated/3)
  Q->pu2 : Gain  Gain=1/(Srated/3)
  RMS{,1..5} (6 alike) : spsRMSLib/RMS  TrueRMS=on  Freq=60  RMSInit=120  Ts=0
  Sqrt : Sqrt
  Sqrt1 : Sqrt
  Sqrt2 : Sqrt
  Subsystem : Subsystem
  Subsystem1 : Subsystem
  Subsystem2 : Subsystem
  Total_Active_Power : Gain
  Total_Apparent_Power : Gain
  Total_RMS_Current : Gain
  Total_Reactive_Power : Gain
  measurements : Outport  VectorParamsAs1DForOutWhenUnconnected=off
  wires:
  [Current_B] -> RMS4/1
  Math Function4/1 -> Add8/1
  [Voltage_A] -> Power Measurement1/1
  [Current_C] -> RMS5/1
  [Current_A] -> Power Measurement1/2
  Sqrt1/1 -> AC_S_2/1  "AC_S_2"
  Math Function1/1 -> Add/2
  Power Measurement1/2 -> AC_Q_1/1
  Math Function5/1 -> Add8/2
  [Voltage_B] -> Power Measurement2/1
  [Current_A] -> RMS3/1
  Power Measurement1/1 -> AC_P_1/1
  [Voltage_C] -> Power Measurement3/1
  Power Measurement2/2 -> AC_Q_2/1
  Add8/1 -> Sqrt2/1
  Power Measurement3/1 -> AC_P_3/1
  [Current_B] -> Power Measurement2/2
  [Q_B] -> Math Function1/1
  PLL (3ph)/1 -> AC_FREQ/1
  [P_B] -> Math Function/1
  [Q_A] -> Math Function3/1
  Sqrt/1 -> AC_S_1/1  "AC_S_1"
  Sqrt2/1 -> AC_S_3/1  "AC_S_3"
  [P_A] -> Math Function2/1
  Add9/1 -> Total_RMS_Current/1
  Math Function3/1 -> Add1/2
  Add1/1 -> Sqrt/1
  Math Function/1 -> Add/1
  Power Measurement3/2 -> AC_Q_3/1
  Math Function2/1 -> Add1/1
  [Current_C] -> Power Measurement3/2
  [P_C] -> Math Function4/1
  [Q_C] -> Math Function5/1
  Add/1 -> Sqrt1/1
  Power Measurement2/1 -> AC_P_2/1
  RAW_MEAS/1 -> Bus Selector/1
  Bus Selector/1 -> [Voltage_A]  "<voltage_pha>"
  Bus Selector/2 -> [Voltage_B]  "<voltage_phb>"
  Bus Selector/3 -> [Voltage_C]  "<voltage_phc>"
  AC_P_2/1 -> Add2/2, Bus Creator2/2  "AC_P_2"
  AC_P_3/1 -> Bus Creator2/3, Add2/3  "AC_P_3"
  Add2/1 -> Total_Active_Power/1
  AC_Q_1/1 -> Bus Creator3/1, Add3/1  "AC_Q_1"
  AC_Q_2/1 -> Bus Creator3/2, Add3/2  "AC_Q_2"
  AC_Q_3/1 -> Bus Creator3/3, Add3/3  "AC_Q_3"
  Add3/1 -> Total_Reactive_Power/1
  Add4/1 -> Total_Apparent_Power/1
  Bus Creator/1 -> [voltage_RMS]
  RMS3/1 -> AC_IRMS_1/1, Add9/1  "AC_IRMS_1"
  RMS4/1 -> AC_IRMS_2/1, Add9/2  "AC_IRMS_2"
  Bus Creator1/1 -> [current_RMS]
  RMS5/1 -> AC_IRMS_3/1, Add9/3  "AC_IRMS_3"
  Total_RMS_Current/1 -> Bus Creator1/4  "Total_RMS_Current"
  Total_Active_Power/1 -> Bus Creator2/4  "Total_Active_Power"
  Bus Creator2/1 -> [active_power]
  Bus Creator3/1 -> [reactive_power]
  Total_Reactive_Power/1 -> Bus Creator3/4  "Total_Reactive_Power"
  [active_power] -> Bus Selector1/1
  Bus Selector1/1 -> [P_A]  "<AC_P_1>"
  Bus Selector1/2 -> [P_B]  "<AC_P_2>"
  Bus Selector1/3 -> [P_C]  "<AC_P_3>"
  [reactive_power] -> Bus Selector2/1
  Bus Creator5/1 -> [apparent_power]
  Total_Apparent_Power/1 -> Bus Creator5/4  "Total_Apparent_Power"
  Bus Selector2/1 -> [Q_A]  "<AC_Q_1>"
  Bus Selector2/2 -> [Q_B]  "<AC_Q_2>"
  Bus Selector2/3 -> [Q_C]  "<AC_Q_3>"
  [voltage_RMS] -> Bus Creator4/1  "voltage_RMS"
  [current_RMS] -> Bus Creator4/2  "current_RMS"
  [frequency] -> Bus Creator4/3  "frequency"
  [reactive_power] -> Bus Creator4/5  "reactive_power"
  Bus Creator4/1 -> measurements/1
  AC_S_1/1 -> Bus Creator5/1, Add4/1
  AC_S_2/1 -> Bus Creator5/2, Add4/2
  AC_S_3/1 -> Bus Creator5/3, Add4/3
  AC_P_1/1 -> Bus Creator2/1, Add2/1  "AC_P_1"
  [Voltage_A] -> Mux/1
  [Voltage_B] -> Mux/2
  [Voltage_C] -> Mux/3
  Mux/1 -> PLL (3ph)/1
  AC_FREQ/1 -> [frequency]  "AC_FREQ"
  Bus Selector/4 -> [Current_A]  "<current_pha>"
  Bus Selector/5 -> [Current_B]  "<current_phb>"
  Bus Selector/6 -> [Current_C]  "<current_phc>"
  [Voltage_C] -> RMS2/1
  [Voltage_B] -> RMS1/1
  [Voltage_A] -> RMS/1
  RMS/1 -> AC_VRMS_1/1  "AC_VRMS_1"
  RMS1/1 -> AC_VRMS_2/1  "AC_VRMS_2"
  RMS2/1 -> AC_VRMS_3/1  "AC_VRMS_3"
  [active_power] -> Bus Creator4/4  "active_power"
  [Q_A] -> Q->pu/1
  [P_A] -> P->pu/1
  P->pu/1 -> Subsystem/1(P)
  Q->pu/1 -> Subsystem/2(Q)
  [P_B] -> P->pu1/1
  [Q_B] -> Q->pu1/1
  [Q_C] -> Q->pu2/1
  [P_C] -> P->pu2/1
  Subsystem/1(PF) -> AC_PF_1/1
  Subsystem1/1(PF) -> AC_PF_2/1
  Subsystem2/1(PF) -> AC_PF_3/1
  AC_PF_1/1 -> Bus Creator6/1
  AC_PF_2/1 -> Bus Creator6/2
  AC_PF_3/1 -> Bus Creator6/3
  Bus Creator6/1 -> [power_factor]  "power_factor"
  [power_factor] -> Bus Creator4/6
  Q->pu1/1 -> Subsystem1/2(Q)
  P->pu1/1 -> Subsystem1/1(P)
  Q->pu2/1 -> Subsystem2/2(Q)
  P->pu2/1 -> Subsystem2/1(P)
  AC_VRMS_1/1 -> Bus Creator/1  "AC_VRMS_1"
  AC_VRMS_2/1 -> Bus Creator/2  "AC_VRMS_2"
  AC_VRMS_3/1 -> Bus Creator/3  "AC_VRMS_3"
  AC_IRMS_1/1 -> Bus Creator1/1  "AC_IRMS_1"
  AC_IRMS_2/1 -> Bus Creator1/2  "AC_IRMS_2"
  AC_IRMS_3/1 -> Bus Creator1/3  "AC_IRMS_3"

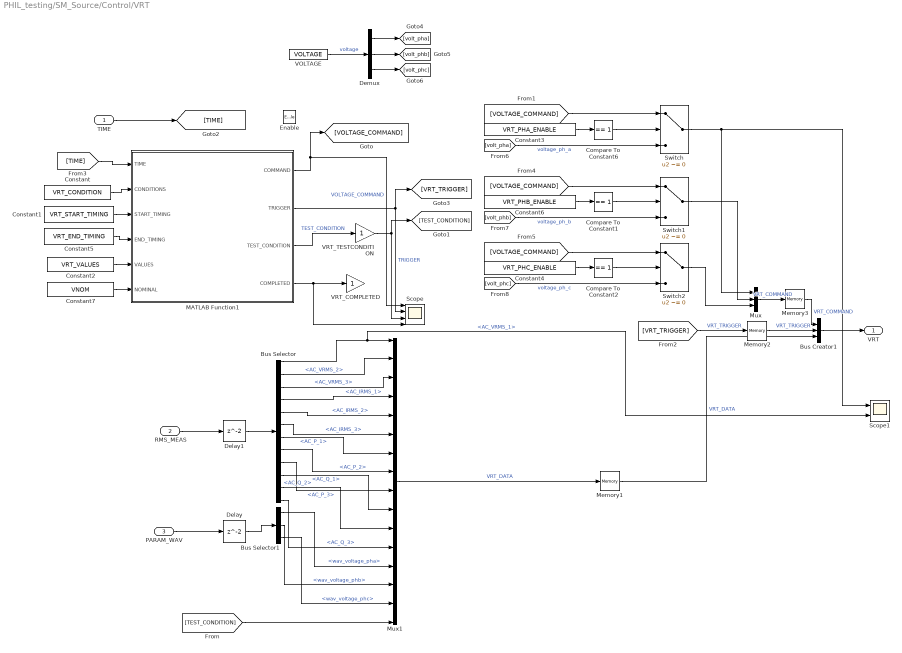
== system PHIL_testing/SM_Source/Control/VRT ==
  TIME : Inport
  RMS_MEAS : Inport  Port=2
  PARAM_WAV : Inport  Port=3
  Enable : EnablePort
  Bus Creator1 : BusCreator  Inputs=3
  Bus Selector : BusSelector  OutputSignals=voltage_RMS.AC_VRMS_1,voltage_RMS.AC_VRMS_2,voltage_RMS.AC_VRMS_3,current_RMS.AC_IRMS_1,current_RMS.AC_IRMS_2,current_RMS.AC_IRMS_3,active_power.AC_P_1,active_power.AC_P_2,active_power.AC_P_3,reactive_power.AC_Q_1,reactive_power.AC_Q_2,reactive_power.AC_Q_3
  Bus Selector1 : BusSelector  OutputSignals=wav_voltage_pha,wav_voltage_phb,wav_voltage_phc
  Compare To Constant1 : simulink/Logic and Bit Operations/Compare To Constant  relop===  const=1  OutDataTypeStr=boolean
  Compare To Constant2 : simulink/Logic and Bit Operations/Compare To Constant  relop===  const=1  OutDataTypeStr=boolean
  Compare To Constant6 : simulink/Logic and Bit Operations/Compare To Constant  relop===  const=1  OutDataTypeStr=boolean
  Constant : Constant  Value=VRT_CONDITION
  Constant1 : Constant  Value=VRT_START_TIMING
  Constant2 : Constant  Value=VRT_VALUES
  Constant3 : Constant  Value=VRT_PHA_ENABLE
  Constant4 : Constant  Value=VRT_PHC_ENABLE
  Constant5 : Constant  Value=VRT_END_TIMING
  Constant6 : Constant  Value=VRT_PHB_ENABLE
  Constant7 : Constant  Value=VNOM
  Delay : Delay
  Delay1 : Delay
  Demux : Demux  Outputs=3
  MATLAB Function1 : MATLAB Function  TreatAsAtomicUnit=on
  Memory1 : Memory  InheritSampleTime=on  LinearizeMemory=on
  Memory2 : Memory  InheritSampleTime=on  LinearizeMemory=on
  Memory3 : Memory  InitialCondition=VNOM  InheritSampleTime=on  LinearizeMemory=on
  Mux : Mux  Inputs=3
  Mux1 : Mux  Inputs=16
  Scope : Scope  NumInputPorts=4
  Scope1 : Scope  NumInputPorts=2
  Switch : Switch  Criteria=u2 ~= 0  SaturateOnIntegerOverflow=off  InputSameDT=off
  Switch1 : Switch  Criteria=u2 ~= 0  SaturateOnIntegerOverflow=off  InputSameDT=off
  Switch2 : Switch  Criteria=u2 ~= 0  SaturateOnIntegerOverflow=off  InputSameDT=off
  VOLTAGE : Constant  Value=VOLTAGE
  VRT_COMPLETED : Gain
  VRT_TESTCONDITION : Gain
  VRT : Outport
  wires:
  Bus Creator1/1 -> VRT/1
  RMS_MEAS/1 -> Delay1/1
  PARAM_WAV/1 -> Delay/1
  Delay/1 -> Bus Selector1/1
  Mux/1 -> Memory3/1  "VRT_COMMAND"
  MATLAB Function1/1(COMMAND) -> Scope/1, [VOLTAGE_COMMAND]  "VOLTAGE_COMMAND"
  Constant2/1 -> MATLAB Function1/5(VALUES)
  Constant1/1 -> MATLAB Function1/3(START_TIMING)
  Constant/1 -> MATLAB Function1/2(CONDITIONS)
  [TIME] -> MATLAB Function1/1(TIME)
  TIME/1 -> [TIME]
  [VRT_TRIGGER] -> Memory2/1  "VRT_TRIGGER"
  Constant5/1 -> MATLAB Function1/4(END_TIMING)
  MATLAB Function1/2(TRIGGER) -> [VRT_TRIGGER], Scope/2  "TRIGGER"
  MATLAB Function1/3(TEST_CONDITION) -> VRT_TESTCONDITION/1  "TEST_CONDITION"
  MATLAB Function1/4(COMPLETED) -> Scope/4, VRT_COMPLETED/1
  [volt_pha] -> Switch/3  "voltage_ph_a"
  [VOLTAGE_COMMAND] -> Switch/1
  Constant3/1 -> Compare To Constant6/1
  Compare To Constant6/1 -> Switch/2
  Compare To Constant1/1 -> Switch1/2
  Constant6/1 -> Compare To Constant1/1
  [VOLTAGE_COMMAND] -> Switch1/1
  [volt_phb] -> Switch1/3  "voltage_ph_b"
  [volt_phc] -> Switch2/3  "voltage_ph_c"
  [VOLTAGE_COMMAND] -> Switch2/1
  Constant4/1 -> Compare To Constant2/1
  Compare To Constant2/1 -> Switch2/2
  Switch/1 -> Scope1/1, Mux/1
  Switch1/1 -> Mux/2
  Switch2/1 -> Mux/3
  Constant7/1 -> MATLAB Function1/6(NOMINAL)
  Mux1/1 -> Memory1/1  "VRT_DATA"
  Delay1/1 -> Bus Selector/1
  Bus Selector/1 -> Scope1/2, Mux1/1  "<AC_VRMS_1>"
  Bus Selector/2 -> Mux1/2  "<AC_VRMS_2>"
  Bus Selector/3 -> Mux1/3  "<AC_VRMS_3>"
  Bus Selector/4 -> Mux1/4  "<AC_IRMS_1>"
  Bus Selector/5 -> Mux1/5  "<AC_IRMS_2>"
  Bus Selector/6 -> Mux1/6  "<AC_IRMS_3>"
  Bus Selector/7 -> Mux1/7  "<AC_P_1>"
  Bus Selector/8 -> Mux1/8  "<AC_P_2>"
  Bus Selector/9 -> Mux1/9  "<AC_P_3>"
  Bus Selector/10 -> Mux1/10  "<AC_Q_1>"
  Bus Selector/11 -> Mux1/11  "<AC_Q_2>"
  Bus Selector/12 -> Mux1/12  "<AC_Q_3>"
  Bus Selector1/1 -> Mux1/13  "<wav_voltage_pha>"
  Bus Selector1/2 -> Mux1/14  "<wav_voltage_phb>"
  Bus Selector1/3 -> Mux1/15  "<wav_voltage_phc>"
  [TEST_CONDITION] -> Mux1/16
  VOLTAGE/1 -> Demux/1  "voltage"
  Demux/1 -> [volt_pha]
  Demux/2 -> [volt_phb]
  Demux/3 -> [volt_phc]
  VRT_TESTCONDITION/1 -> [TEST_CONDITION], Scope/3
  Memory1/1 -> Bus Creator1/3  "VRT_DATA"
  Memory2/1 -> Bus Creator1/2  "VRT_TRIGGER"
  Memory3/1 -> Bus Creator1/1  "VRT_COMMAND"
